simulink model "model_open_loop_test"  (R2017a)
settings: Solver=VariableStepAuto  StartTime=0.0  StopTime=10  FixedStep=1/(1000000e3)  RelTol=1e-3
values from neighbouring files (symbols this model uses):
  motor = gm9434    [motor_code.m]
undefined symbols (not defined in the file or in its folder): current_ctrl
libraries: simulink x1
settings Model: Creator=rodrigo  LastModifiedBy=rodrigo

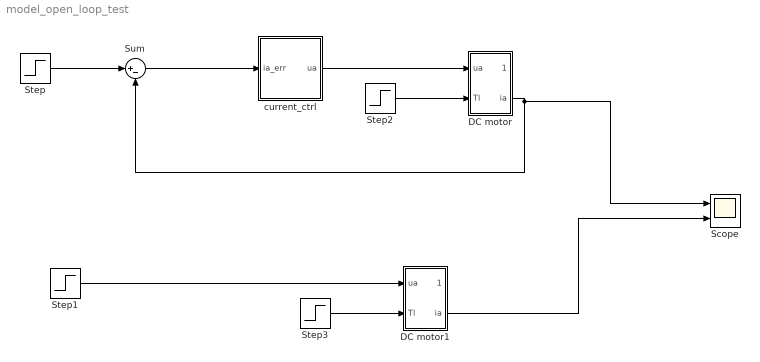
== system model_open_loop_test ==
  DC motor : Subsystem
  DC motor1 : Subsystem
  Scope : Scope  NumInputPorts=2
  Step : Step  After=0.2957  SampleTime=0
  Step1 : Step  After=12  SampleTime=0
  Step2 : Step  After=0.01  SampleTime=0
  Step3 : Step  After=0.01  SampleTime=0
  Sum : Sum  Inputs=|+-
  current_ctrl : Subsystem
  wires:
  current_ctrl/1(ua) -> DC motor/1(ua)
  Step2/1 -> DC motor/2(Tl)
  Sum/1 -> current_ctrl/1(ia_err)
  DC motor/2(ia) -> Scope/1, Sum/2
  Step/1 -> Sum/1
  Step3/1 -> DC motor1/2(Tl)
  Step1/1 -> DC motor1/1(ua)
  DC motor1/2(ia) -> Scope/2

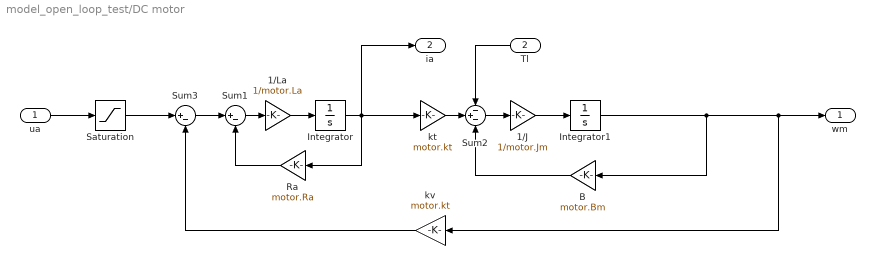
== system model_open_loop_test/DC motor ==
  ua : Inport
  Tl : Inport  Port=2
  1/J : Gain  Gain=1/motor.Jm
  1/La : Gain  Gain=1/motor.La
  B : Gain  Gain=motor.Bm
  Integrator : Integrator  ZeroCross=off
  Integrator1 : Integrator
  Ra : Gain  Gain=motor.Ra
  Saturation : Saturate  UpperLimit=12  LowerLimit=-12
  Sum1 : Sum  Inputs=|+-
  Sum2 : Sum  Inputs=-+-
  Sum3 : Sum  Inputs=|+-
  kt : Gain  Gain=motor.kt
  kv : Gain  Gain=motor.kt
  wm : Outport
  ia : Outport  Port=2
  wires:
  1/J/1 -> Integrator1/1
  Sum2/1 -> 1/J/1
  Integrator1/1 -> B/1, wm/1, kv/1
  ua/1 -> Saturation/1
  Integrator/1 -> kt/1, Ra/1, ia/1
  Ra/1 -> Sum1/2
  1/La/1 -> Integrator/1
  Tl/1 -> Sum2/1
  kv/1 -> Sum3/2
  Sum3/1 -> Sum1/1
  kt/1 -> Sum2/2
  Sum1/1 -> 1/La/1
  Saturation/1 -> Sum3/1
  B/1 -> Sum2/3

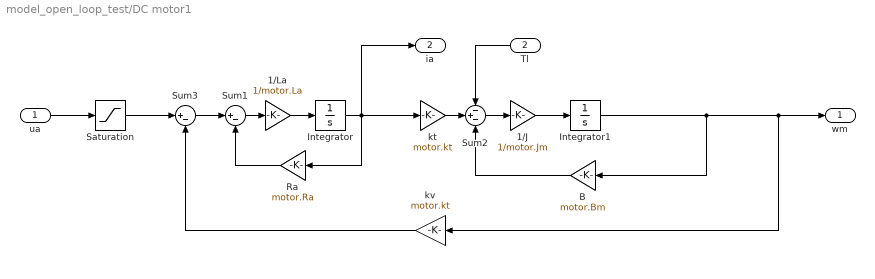
== system model_open_loop_test/DC motor1 ==
  ua : Inport
  Tl : Inport  Port=2
  1/J : Gain  Gain=1/motor.Jm
  1/La : Gain  Gain=1/motor.La
  B : Gain  Gain=motor.Bm
  Integrator : Integrator  ZeroCross=off
  Integrator1 : Integrator
  Ra : Gain  Gain=motor.Ra
  Saturation : Saturate  UpperLimit=12  LowerLimit=-12
  Sum1 : Sum  Inputs=|+-
  Sum2 : Sum  Inputs=-+-
  Sum3 : Sum  Inputs=|+-
  kt : Gain  Gain=motor.kt
  kv : Gain  Gain=motor.kt
  wm : Outport
  ia : Outport  Port=2
  wires:
  1/J/1 -> Integrator1/1
  Sum2/1 -> 1/J/1
  Integrator1/1 -> B/1, wm/1, kv/1
  ua/1 -> Saturation/1
  Integrator/1 -> kt/1, Ra/1, ia/1
  Ra/1 -> Sum1/2
  1/La/1 -> Integrator/1
  Tl/1 -> Sum2/1
  kv/1 -> Sum3/2
  Sum3/1 -> Sum1/1
  kt/1 -> Sum2/2
  Sum1/1 -> 1/La/1
  Saturation/1 -> Sum3/1
  B/1 -> Sum2/3

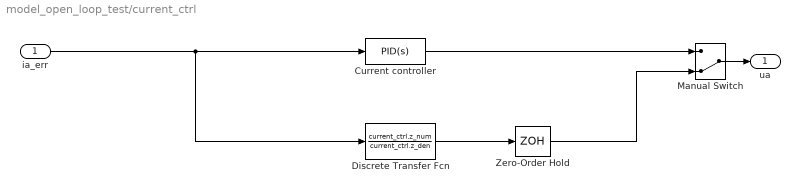
== system model_open_loop_test/current_ctrl ==
  ia_err : Inport
  Current controller : simulink/Continuous/PID Controller  Controller=PID  TimeDomain=Continuous-time  SampleTime=-1  IntegratorMethod=Forward Euler  FilterMethod=Forward Euler  Form=Parallel  UseFilter=off  ControllerParametersSource=internal  P=current_ctrl.kp  I=current_ctrl.ki  D=0  N=100  InitialConditionSource=internal  InitialConditionForIntegrator=0  InitialConditionForFilter=0  ExternalReset=none  ZeroCross=off  LimitOutput=off  UpperSaturationLimit=12  LowerSaturationLimit=-12  LinearizeAsGain=off  AntiWindupMode=back-calculation  Kb=1  TrackingMode=off  Kt=1  PParamMin=[]  PParamMax=[]  IParamMin=[]  IParamMax=[]  DParamMin=[]  DParamMax=[]  NParamMin=[]  NParamMax=[]  KbParamMin=[]  KbParamMax=[]  KtParamMin=[]  KtParamMax=[]  POutMin=[]  POutMax=[]  IOutMin=[]  IOutMax=[]  DOutMin=[]  DOutMax=[]  NOutMin=[]  NOutMax=[]  KbOutMin=[]  KbOutMax=[]  KtOutMin=[]  KtOutMax=[]  IntegratorOutMin=[]  IntegratorOutMax=[]  FilterOutMin=[]  FilterOutMax=[]  SumOutMin=[]  SumOutMax=[]  SumI1OutMin=[]  SumI1OutMax=[]  SumI2OutMin=[]  SumI2OutMax=[]  SumI3OutMin=[]  SumI3OutMax=[]  SumDOutMin=[]  SumDOutMax=[]  SaturationOutMin=[]  SaturationOutMax=[]  IntegratorContinuousStateAttributes=''  IntegratorStateMustResolveToSignalObject=off  IntegratorRTWStateStorageClass=Auto  FilterContinuousStateAttributes=''  FilterStateMustResolveToSignalObject=off  FilterRTWStateStorageClass=Auto  DifferentiatorICPrevScaledInput=0  DifferentiatorOutMin=[]  DifferentiatorOutMax=[]  InitialConditionSetting=State (most efficient)
  Discrete Transfer Fcn : DiscreteTransferFcn  Numerator=current_ctrl.z_num  Denominator=current_ctrl.z_den  SampleTime=current_ctrl.Ts
  Manual Switch : ManualSwitch  CurrentSetting=0
  Zero-Order Hold : ZeroOrderHold  SampleTime=current_ctrl.Ts
  ua : Outport
  wires:
  ia_err/1 -> Discrete Transfer Fcn/1, Current controller/1
  Current controller/1 -> Manual Switch/1
  Discrete Transfer Fcn/1 -> Zero-Order Hold/1
  Zero-Order Hold/1 -> Manual Switch/2
  Manual Switch/1 -> ua/1
